simulink model "untitled"  (R2023a)
settings: Solver=VariableStepAuto  StartTime=0.0  StopTime=tf  MaxStep=maxstep  RelTol=tol1
values from neighbouring files (symbols this model uses):
  C = 1e-5    (= 1e-05)    [Problem2_lab03.m]    (also in script1.m)
  R = 2000    [Problem2_lab03.m]    (also in script1.m)
settings Model: Creator=mcconncm  LastModifiedBy=mcconncm

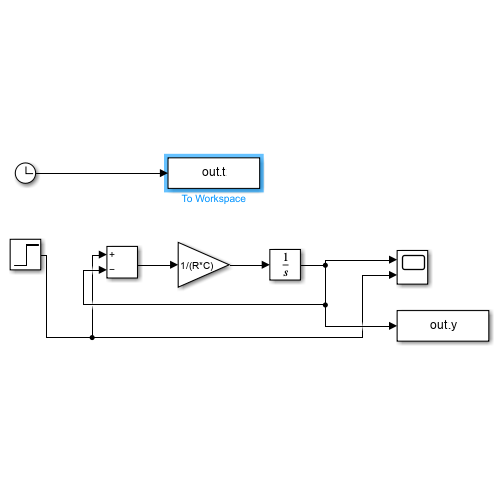
[thumbnail: Simulink's stored preview of the top-level diagram]
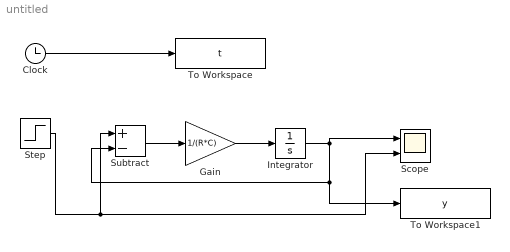
== system untitled ==
  Clock : Clock
  Gain : Gain  Gain=1/(R*C)
  Integrator : Integrator
  Scope : Scope  NumInputPorts=2
  Step : Step  Time=0  SampleTime=0
  Subtract : Sum  Inputs=+-
  To Workspace : ToWorkspace  VariableName=t  SampleTime=-1
  To Workspace1 : ToWorkspace  VariableName=y  SampleTime=-1
  wires:
  Gain/1 -> Integrator/1
  Subtract/1 -> Gain/1
  Integrator/1 -> Scope/1, To Workspace1/1, Subtract/2
  Step/1 -> Scope/2, Subtract/1
  Clock/1 -> To Workspace/1
